simulink model "middle_new"  (R2014a)
settings: Solver=FixedStepDiscrete  StartTime=0.0  StopTime=SimLength  FixedStep=0.01  RelTol=1e-3
settings Model: Creator=Maik  LastModifiedBy=Jonas

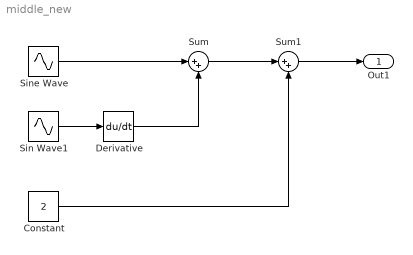
== system middle_new ==
  Constant : Constant  Value=2
  Derivative : Derivative
  Sin Wave1 : Sin  Amplitude=0.4  Frequency=sqrt(3)
  Sine Wave : Sin  Frequency=0.5
  Sum : Sum  Inputs=|++
  Sum1 : Sum  Inputs=|++
  Out1 : Outport
  wires:
  Sin Wave1/1 -> Derivative/1
  Sine Wave/1 -> Sum/1
  Derivative/1 -> Sum/2
  Sum/1 -> Sum1/1
  Constant/1 -> Sum1/2
  Sum1/1 -> Out1/1
